simulink model "systema_script"  (R2019a)
settings: Solver=ode4  StartTime=0.0  StopTime=20  FixedStep=0.01  RelTol=1e-3  EnableMultiTasking=on
undefined symbols (not defined in the file or in its folder): dfod, DiscIntNeverNeededParam, f_enable, gain, i_enable, iokd, ioki, iokp, Kd, Kp, Lambda
libraries: simulink x9
settings Model: Creator=ece  LastModifiedBy=standard
settings DataIOCC: SaveFormat=Array  ReturnWorkspaceOutputs=off  SignalLoggingName=sigsOut
settings OptimizationCC: OptimizeBlockIOStorage=off  BufferReuse=off  GlobalBufferReuse=off  ExpressionFolding=off  ExpressionDepthLimit=2147483647  LocalBlockOutputs=off  InitFltsAndDblsToZero=on  LifeSpan=inf  OptimizeDataStoreBuffers=off  BusAssignmentInplaceUpdate=off
settings DebuggingCC: SaveWithParameterizedLinksMsg=none  UnderspecifiedInitializationDetection=Classic  MergeDetectMultiDrivingBlocksExec=none  SignalResolutionControl=TryResolveAllWithWarning  MultiTaskDSMMsg=warning  MultiTaskCondExecSysMsg=none  FcnCallInpInsideContextMsg=warning  StateNameClashWarn=warning  PregeneratedLibrarySubsystemCodeDiagnostic=none  SFUnexpectedBacktrackingDiag=warning  SFNoUnconditionalDefaultTransitionDiag=warning  SFExecutionAtInitializationDiag=none  ArithmeticOperatorsInVariantConditions=warning
settings HardwareCC: ProdBitPerPointer=32  ProdBitPerSizeT=32  ProdBitPerPtrDiffT=32  ProdLargestAtomicFloat=None  ProdIntDivRoundTo=Undefined  ProdEndianess=Unspecified  ProdWordSize=32  ProdHWDeviceType=32-bit Generic  TargetUnknown=on
settings ModelReferenceCC: PropagateSignalLabelsOutOfModel=off
settings SFSimCC: SimUseLocalCustomCode=off
settings RTWCC: RTWUseLocalCustomCode=off
settings CodeAppCC: StateflowObjectComments=on
settings GRTTargetCC: TargetFcnLib=ansi_tfl_tmw.mat  TargetLangStandard=C89/C90 (ANSI)  ModelReferenceCompliant=off  GeneratePreprocessorConditionals=Disable all  CombineOutputUpdateFcns=off  MatFileLogging=off  GRTInterface=on
settings ConfigComp: CovMetricSettings=dw  CovHtmlReporting=on  CovSaveCumulativeToWorkspaceVar=on  CovSaveSingleToWorkspaceVar=on  CovExternalEMLEnable=off

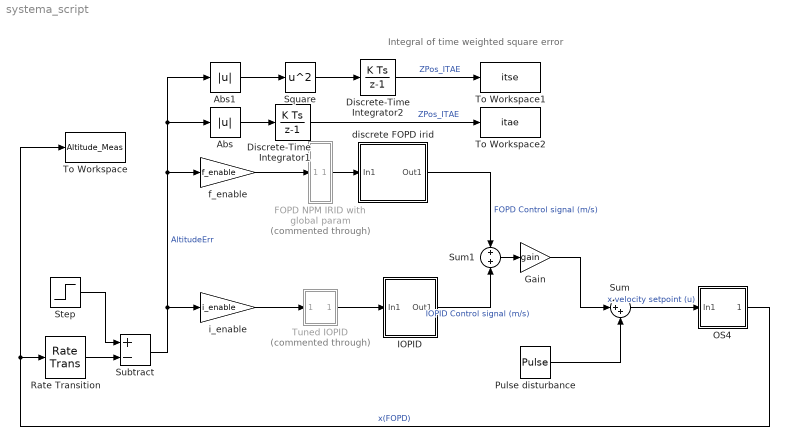
== system systema_script ==
  note: Integral of time weighted square error
  Abs : Abs
  Abs1 : Abs
  Discrete-Time Integrator1 : DiscreteIntegrator  SampleTime=-1  ICPrevOutput=DiscIntNeverNeededParam  ICPrevScaledInput=DiscIntNeverNeededParam
  Discrete-Time Integrator2 : DiscreteIntegrator  SampleTime=-1  ICPrevOutput=DiscIntNeverNeededParam  ICPrevScaledInput=DiscIntNeverNeededParam
  FOPD NPM IRID with global param : Subsystem  Commented=through
  Gain : Gain  Gain=gain
  IOPID : Subsystem
  OS4 : Subsystem
  Pulse disturbance : DiscretePulseGenerator  PulseType=Time based  Amplitude=0  Period=20  PhaseDelay=1
  Rate Transition : RateTransition  OutPortSampleTime=0.01
  Square : Math  Operator=square  SaturateOnIntegerOverflow=on
  Step : Step  Time=5  SampleTime=0.01
  Subtract : Sum  Inputs=+-
  Sum : Sum  Inputs=|++
  Sum1 : Sum  Inputs=+|+
  To Workspace : ToWorkspace  VariableName=Altitude_Meas  SaveFormat=Timeseries  SampleTime=-1
  To Workspace1 : ToWorkspace  VariableName=itse  SaveFormat=Timeseries  SampleTime=-1
  To Workspace2 : ToWorkspace  VariableName=itae  SaveFormat=Timeseries  SampleTime=-1
  Tuned IOPID : Subsystem  Commented=through
  discrete FOPD irid : Subsystem
  f_enable : Gain  Gain=f_enable
  i_enable : Gain  Gain=i_enable
  wires:
  IOPID/1(Out1) -> Sum1/2  "IOPID Control signal (m/s)"
  OS4/1(Out4) -> Rate Transition/1, To Workspace/1  "x(FOPD)"
  Step/1 -> Subtract/1
  discrete FOPD irid/1(Out1) -> Sum1/1  "FOPD Control signal (m/s)"
  Rate Transition/1 -> Subtract/2
  Pulse disturbance/1 -> Sum/2
  Sum/1 -> OS4/1(In1)  "x velocity setpoint (u)"
  Sum1/1 -> Gain/1
  f_enable/1 -> FOPD NPM IRID with global param/1(In1)
  i_enable/1 -> Tuned IOPID/1(In1)
  Gain/1 -> Sum/1
  Abs1/1 -> Square/1
  Subtract/1 -> i_enable/1, Abs/1, Abs1/1, f_enable/1  "AltitudeErr"
  Abs/1 -> Discrete-Time Integrator1/1
  Discrete-Time Integrator1/1 -> To Workspace2/1  "ZPos_ITAE"
  Square/1 -> Discrete-Time Integrator2/1
  Discrete-Time Integrator2/1 -> To Workspace1/1  "ZPos_ITAE"
  Tuned IOPID/1(Out1) -> IOPID/1(In1)
  FOPD NPM IRID with global param/1(Out1) -> discrete FOPD irid/1(In1)

== system systema_script/FOPD NPM IRID with global param ==
  note: FOPD controller
  In1 : Inport
  Discrete Transfer Fcn : DiscreteTransferFcn  Commented=through  Numerator=dfod.Num{1,1}  Denominator=dfod.Denominator{1,1}  SampleTime=0.01
  "Fractional operator " : Subsystem  Commented=through  mask{gam=Lambda, ww=[1e-3, 1e3], n=5, kF1=on, kF=Modified Oustaloup filter}
      mask prompts: gam "Derivative order gamma"; ww "Frequency range [wb,wh]"; n "Apprixmation order"; kF1 "Is a low-pass filter required?"; kF "Filter type"
      mask init:
      | wb=ww(1); wh=ww(2); 
      | if kF==1, G=ousta_fod(gam,n,wb,wh);
      | else, G=new_fod(gam,n,wb,wh); end
      | num=G.num{1}; den=G.den{1}; T=1/wh; str='Fractional\n';
      | if isnumeric(gam)
      | 	if gam>0, str=[str, 'Der  s^' num2str(gam) ];
      | 	else, str=[str, 'Int  s^{' num2str(gam) '}']; end
      | else, str=[str, 'Der  s^gam']; end
      | if kF1==1, G=G*tf(1,[T 1]); end
      mask TypeOptions kF: Oustaloup filter | Modified Oustaloup filter | Matsuda-Fujii filter
      mask Display: disp(str)
  Saturation : Saturate  UpperLimit=5  LowerLimit=-5
  Saturation1 : Saturate  UpperLimit=5  LowerLimit=-5
  Sum : Sum  Inputs=++|
  k_d : Gain  Gain=Kd
  k_p : Gain  Gain=Kp
  Out1 : Outport
  wires:
  In1/1 -> k_p/1  "P"
  Sum/1 -> Saturation1/1
  Saturation1/1 -> Out1/1
  k_d/1 -> "Fractional operator "/1(In1)  "DD_input"
  Discrete Transfer Fcn/1 -> Saturation/1  "DD_out"
  Saturation/1 -> Sum/2  "D"
  "Fractional operator "/1(Out1) -> Discrete Transfer Fcn/1
  k_p/1 -> Sum/1, k_d/1  "DD_input"

== system systema_script/IOPID ==
  In1 : Inport
  Discrete Derivative : simulink/Discrete/Discrete Derivative  gainval=1.0  ICPrevScaledInput=0.0  OutMin=[]  OutMax=[]  OutDataType=fixdt(1, 16)  OutScaling=2^-10  DoSatur=off
  Discrete-Time Integrator : DiscreteIntegrator  SampleTime=-1  ICPrevOutput=DiscIntNeverNeededParam  ICPrevScaledInput=DiscIntNeverNeededParam
  Gain : Gain  Gain=1.58
  Gain1 : Gain  Gain=0.182
  Gain2 : Gain  Gain=1.49
  Sum2 : Sum  Inputs=+++
  Out1 : Outport
  wires:
  In1/1 -> Gain/1, Gain2/1, Gain1/1
  Gain/1 -> Sum2/1
  Gain1/1 -> Discrete-Time Integrator/1
  Gain2/1 -> Discrete Derivative/1
  Sum2/1 -> Out1/1
  Discrete Derivative/1 -> Sum2/3
  Discrete-Time Integrator/1 -> Sum2/2

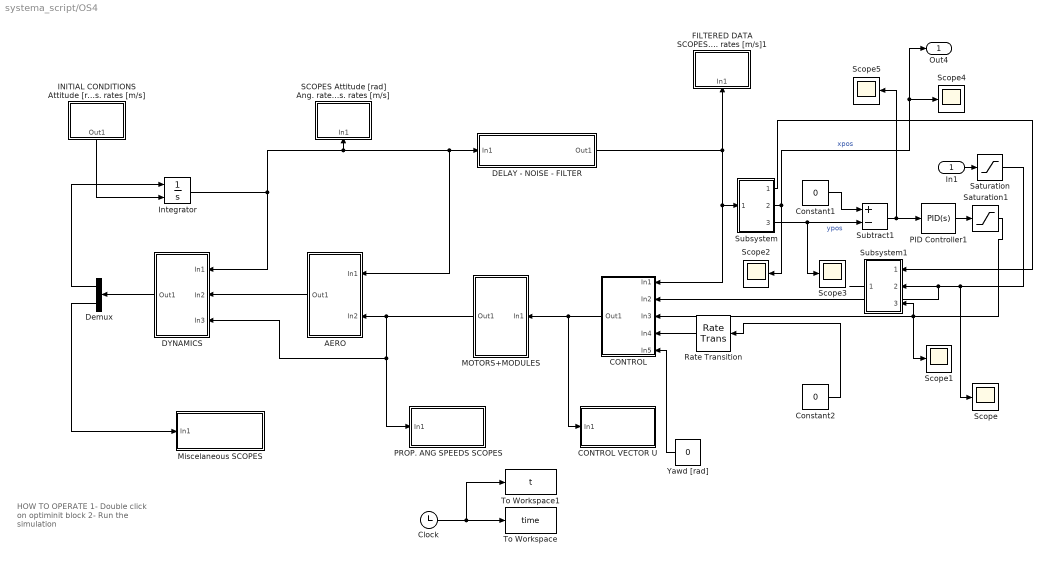
== system systema_script/OS4 ==
  note: HOW TO OPERATE
      | 1- Double click on optiminit block
      | 2- Run the simulation
  In1 : Inport
  AERO : Subsystem
  CONTROL : Subsystem
  CONTROL VECTOR U : Subsystem
  Clock : Clock
  Constant1 : Constant  Value=0
  Constant2 : Constant  Value=0
  DELAY - NOISE - FILTER : Subsystem
  DYNAMICS : Subsystem
  Demux : Demux  Outputs=2
  FILTERED DATA SCOPES Attitude [rad] Ang. rates [rad/sec] position [m] Pos. rates [m/s]1 : Subsystem
  "INITIAL CONDITIONS Attitude [rad] Ang. rates [rad/sec] position [m] Pos. rates [m/s] " : Subsystem
  Integrator : Integrator  InitialConditionSource=external
  MOTORS+MODULES : Subsystem
  Miscelaneous SCOPES : Subsystem
  PID Controller1 : simulink/Continuous/PID Controller  Controller=PID  Form=Parallel  TimeDomain=Continuous-time  SampleTime=-1  IntegratorMethod=Forward Euler  FilterMethod=Forward Euler  ControllerParametersSource=internal  P=1  I=0.2  D=0  UseFilter=on  N=100  TunerSelectOption=Transfer Function Based (PID Tuner App)  InitialConditionSource=internal  InitialConditionForIntegrator=0  InitialConditionForFilter=0  DifferentiatorICPrevScaledInput=0  ExternalReset=none  TrackingMode=off  Kt=1  LimitOutput=off  UpperSaturationLimit=inf  LowerSaturationLimit=-inf  LinearizeAsGain=off  AntiWindupMode=none  Kb=1  POutMin=[]  POutMax=[]  IOutMin=[]  IOutMax=[]  DOutMin=[]  DOutMax=[]  NOutMin=[]  NOutMax=[]  SumOutMin=[]  SumOutMax=[]  SaturationOutMin=[]  SaturationOutMax=[]  PParamMin=[]  PParamMax=[]  IParamMin=[]  IParamMax=[]  DParamMin=[]  DParamMax=[]  NParamMin=[]  NParamMax=[]  KbParamMin=[]  KbParamMax=[]  KtParamMin=[]  KtParamMax=[]  KbOutMin=[]  KbOutMax=[]  KtOutMin=[]  KtOutMax=[]  IntegratorOutMin=[]  IntegratorOutMax=[]  FilterOutMin=[]  FilterOutMax=[]  SumI1OutMin=[]  SumI1OutMax=[]  SumI2OutMin=[]  SumI2OutMax=[]  SumI3OutMin=[]  SumI3OutMax=[]  SumI4OutMin=[]  SumI4OutMax=[]  SumDOutMin=[]  SumDOutMax=[]  DifferentiatorOutMin=[]  DifferentiatorOutMax=[]  FilterDiffOutCoefMin=[]  FilterDiffOutCoefMax=[]  ReciprocalOutMin=[]  ReciprocalOutMax=[]  SumDenOutMin=[]  SumDenOutMax=[]  SumNumOutMin=[]  SumNumOutMax=[]  DivideOutMin=[]  DivideOutMax=[]  IntegratorContinuousStateAttributes=''  IntegratorStateMustResolveToSignalObject=off  IntegratorRTWStateStorageClass=Auto  FilterContinuousStateAttributes=''  FilterStateMustResolveToSignalObject=off  FilterRTWStateStorageClass=Auto  ParallelPVariant=InternalParameters  IdealPVariant=Disabled  IVariant=InternalParameters  DVariant=InternalParameters  IntegratorVariant=Continuous  SatVariant=Disabled  AWVariant=Passthrough  PCopyVariant=Disabled  TRVariant=Disabled  FdbkBlocksVariant=Forward  IdealPFdbkVariant=Disabled  SatFdbkVariant=Disabled  DerivativeFilterVariant=ContFilter  NVariant=InternalParameters  NCopyVariant=Disabled  FilterICVariant=InternalICsFilter  IntegratorICVariant=InternalICs  ExternalResetVariant=Disabled  TRSumVariant=Passthrough  SumFdbkVariant=Disabled  SumVariant=Sum_PID
  PROP. ANG SPEEDS SCOPES : Subsystem
  Rate Transition : RateTransition
  SCOPES Attitude [rad] Ang. rates [rad/sec] position [m] Pos. rates [m/s] : Subsystem
  Saturation : Saturate  UpperLimit=20  LowerLimit=-20
  Saturation1 : Saturate  UpperLimit=20  LowerLimit=-20
  Scope{,1..5} (6 alike) : Scope
  Subsystem : Subsystem
  Subsystem1 : Subsystem
  Subtract1 : Sum  Inputs=+-
  To Workspace : ToWorkspace  VariableName=time  SampleTime=-1
  To Workspace1 : ToWorkspace  VariableName=t  SampleTime=-1
  Yawd [rad] : Constant  Value=0
  Out4 : Outport
  wires:
  Demux/2 -> Miscelaneous SCOPES/1(In1)
  Integrator/1 -> SCOPES Attitude [rad] Ang. rates [rad/sec] position [m] Pos. rates [m/s]/1(In1), DELAY - NOISE - FILTER/1(In1), AERO/1(In1), DYNAMICS/1(In1)
  MOTORS+MODULES/1(Out1) -> AERO/2(In2), DYNAMICS/3(In3), PROP. ANG SPEEDS SCOPES/1(In1)
  Rate Transition/1 -> CONTROL/4(In4)
  CONTROL/1(Out1) -> MOTORS+MODULES/1(In1), CONTROL VECTOR U/1(In1)
  Yawd [rad]/1 -> CONTROL/5(In5)
  Constant2/1 -> Rate Transition/1
  Subsystem/2(Out3) -> Out4/1, Scope4/1, Scope2/1  "xpos"
  DELAY - NOISE - FILTER/1(Out1) -> FILTERED DATA SCOPES Attitude [rad] Ang. rates [rad/sec] position [m] Pos. rates [m/s]1/1(In1), CONTROL/1(In1), Subsystem/1(In1)
  Saturation1/1 -> CONTROL/3(In3), Subsystem1/3(In3), Scope1/1
  Saturation/1 -> Scope/1, Subsystem1/2(In2), CONTROL/2(In2)
  Subtract1/1 -> PID Controller1/1, Scope5/1
  Constant1/1 -> Subtract1/1
  Subsystem/1(Out2) -> Subsystem1/1(In1)
  PID Controller1/1 -> Saturation1/1
  Subsystem1/1(Out5) -> ?
  Subsystem/3(Out4) -> Subtract1/2, Scope3/1  "ypos"
  DYNAMICS/1(Out1) -> Demux/1
  In1/1 -> Saturation/1
  AERO/1(Out1) -> DYNAMICS/2(In2)
  "INITIAL CONDITIONS Attitude [rad] Ang. rates [rad/sec] position [m] Pos. rates [m/s] "/1(Out1) -> Integrator/2
  Clock/1 -> To Workspace/1, To Workspace1/1
  Demux/1 -> Integrator/1

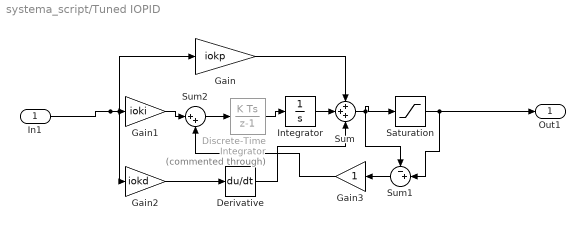
== system systema_script/Tuned IOPID ==
  In1 : Inport
  Derivative : Derivative
  Discrete-Time Integrator : DiscreteIntegrator  Commented=through  SampleTime=-1  ICPrevOutput=DiscIntNeverNeededParam  ICPrevScaledInput=DiscIntNeverNeededParam
  Gain : Gain  Gain=iokp
  Gain1 : Gain  Gain=ioki
  Gain2 : Gain  Gain=iokd
  Gain3 : Gain
  Integrator : Integrator
  Saturation : Saturate  UpperLimit=10  LowerLimit=-10
  Sum : Sum  Inputs=+++
  Sum1 : Sum  Inputs=-+|
  Sum2 : Sum  Inputs=|++
  Out1 : Outport
  wires:
  Sum/1 -> Saturation/1, Sum1/1
  Sum1/1 -> Gain3/1
  In1/1 -> Gain2/1, Gain/1, Gain1/1
  Sum2/1 -> Discrete-Time Integrator/1
  Derivative/1 -> Sum/3
  Gain/1 -> Sum/1
  Discrete-Time Integrator/1 -> Integrator/1
  Gain1/1 -> Sum2/1
  Gain3/1 -> Sum2/2
  Gain2/1 -> Derivative/1
  Saturation/1 -> Sum1/2, Out1/1
  Integrator/1 -> Sum/2

== system systema_script/discrete FOPD irid ==
  In1 : Inport
  Discrete Transfer Fcn : DiscreteTransferFcn  Numerator=[1,-3.83915008336134,5.68830152517571,-4.01123857485582,1.31417664909109,-0.152089532241851]  Denominator=[8.08505564819526e-05,-0.000204449367025327,0.000263365621479140,-0.000214834792194125,8.91860440440781e-05,-1.22283037538058e-05]
  Discrete-Time Integrator : DiscreteIntegrator  SampleTime=-1  ICPrevOutput=DiscIntNeverNeededParam  ICPrevScaledInput=DiscIntNeverNeededParam
  Gain : Gain  Gain=1.5489
  Gain1 : Gain  Gain=0.8829
  Sum : Sum  Inputs=|++
  Out1 : Outport
  wires:
  Sum/1 -> Out1/1  "vx set"
  In1/1 -> Gain/1  "x err"
  Gain/1 -> Gain1/1, Sum/1
  Gain1/1 -> Discrete Transfer Fcn/1
  Discrete Transfer Fcn/1 -> Discrete-Time Integrator/1
  Discrete-Time Integrator/1 -> Sum/2

== system systema_script/FOPD NPM IRID with global param/Fractional operator  ==
  In1 : Inport
  Transfer Fcn : TransferFcn  Numerator=num  Denominator=den
  Out1 : Outport
  wires:
  In1/1 -> Transfer Fcn/1
  Transfer Fcn/1 -> Out1/1

== system systema_script/OS4/AERO ==
  In1 : Inport
  In2 : Inport  Port=2
  AERO Attitude [rad] : MATLABFcn  MATLABFcn=aero  OutputDimensions=24
  Mux1 : Mux  Inputs=2
  Out1 : Outport
  wires:
  In1/1 -> Mux1/1
  In2/1 -> Mux1/2
  Mux1/1 -> AERO Attitude [rad]/1
  AERO Attitude [rad]/1 -> Out1/1

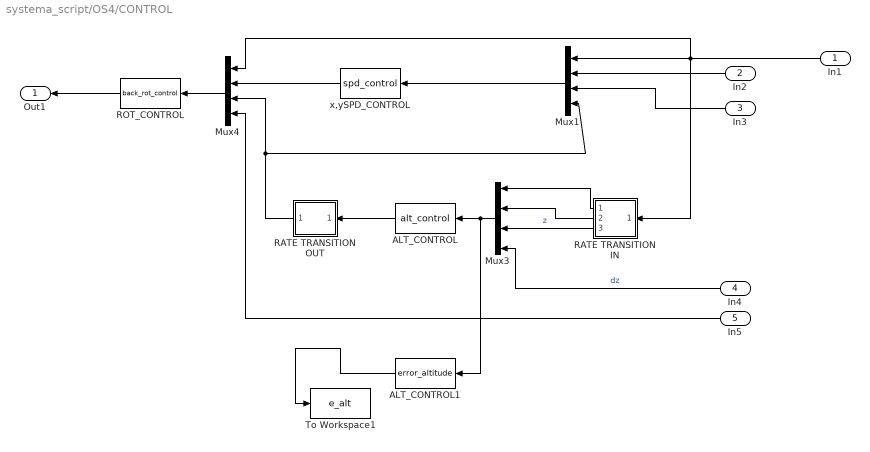
== system systema_script/OS4/CONTROL ==
  In1 : Inport
  In2 : Inport  Port=2
  In3 : Inport  Port=3
  In4 : Inport  Port=4
  In5 : Inport  Port=5
  ALT_CONTROL : MATLABFcn  MATLABFcn=alt_control  OutputDimensions=1  SampleTime=0.05
  ALT_CONTROL1 : MATLABFcn  MATLABFcn=error_altitude  OutputDimensions=1  SampleTime=0.05
  Mux1 : Mux
  Mux3 : Mux
  Mux4 : Mux
  RATE TRANSITION IN : Subsystem
  RATE TRANSITION OUT : Subsystem
  ROT_CONTROL : MATLABFcn  MATLABFcn=back_rot_control  OutputDimensions=6
  To Workspace1 : ToWorkspace  VariableName=e_alt  SampleTime=-1
  x,ySPD_CONTROL : MATLABFcn  MATLABFcn=spd_control  OutputDimensions=2
  Out1 : Outport
  wires:
  Mux1/1 -> x,ySPD_CONTROL/1
  ROT_CONTROL/1 -> Out1/1
  In1/1 -> Mux1/1, RATE TRANSITION IN/1(In1), Mux4/1
  In2/1 -> Mux1/2
  x,ySPD_CONTROL/1 -> Mux4/2
  Mux4/1 -> ROT_CONTROL/1
  ALT_CONTROL/1 -> RATE TRANSITION OUT/1(In1)
  In5/1 -> Mux4/4
  RATE TRANSITION OUT/1(Out1) -> Mux4/3, Mux1/4
  Mux3/1 -> ALT_CONTROL/1, ALT_CONTROL1/1
  RATE TRANSITION IN/1(Out1) -> Mux3/1
  RATE TRANSITION IN/2(Out2) -> Mux3/2
  RATE TRANSITION IN/3(Out3) -> Mux3/3  "z"
  In4/1 -> Mux3/4  "dz"
  In3/1 -> Mux1/3
  ALT_CONTROL1/1 -> To Workspace1/1

== system systema_script/OS4/CONTROL VECTOR U ==
  In1 : Inport
  Demux1 : Demux  Outputs=6
  U{1..4} (4 alike) : Scope
  e1 : Scope
  e2 : Scope
  wires:
  In1/1 -> Demux1/1
  Demux1/4 -> U4/1
  Demux1/3 -> U3/1
  Demux1/2 -> U2/1
  Demux1/1 -> U1/1
  Demux1/5 -> e1/1
  Demux1/6 -> e2/1

== system systema_script/OS4/DELAY - NOISE - FILTER ==
  In1 : Inport
  DELAYS : Subsystem
  LP FILTER : MATLABFcn  MATLABFcn=sam5_filter  OutputDimensions=12  OutputSignalType=real
  NOISY DATA SCOPES Attitude [rad] Ang. rates [rad/sec] position [m] Pos. rates [m/s]1 : Subsystem
  W. NORMAL NOISE1 : Subsystem
  Out1 : Outport
  wires:
  In1/1 -> DELAYS/1(In1)
  DELAYS/1(Out1) -> NOISY DATA SCOPES Attitude [rad] Ang. rates [rad/sec] position [m] Pos. rates [m/s]1/1(In1), LP FILTER/1
  LP FILTER/1 -> Out1/1

== system systema_script/OS4/DYNAMICS ==
  In1 : Inport
  In2 : Inport  Port=2
  In3 : Inport  Port=3
  DYNAMICS : MATLABFcn  MATLABFcn=dinamica  OutputDimensions=18
  Mux1 : Mux  Inputs=3
  Out1 : Outport
  wires:
  DYNAMICS/1 -> Out1/1
  Mux1/1 -> DYNAMICS/1
  In2/1 -> Mux1/2
  In1/1 -> Mux1/1
  In3/1 -> Mux1/3

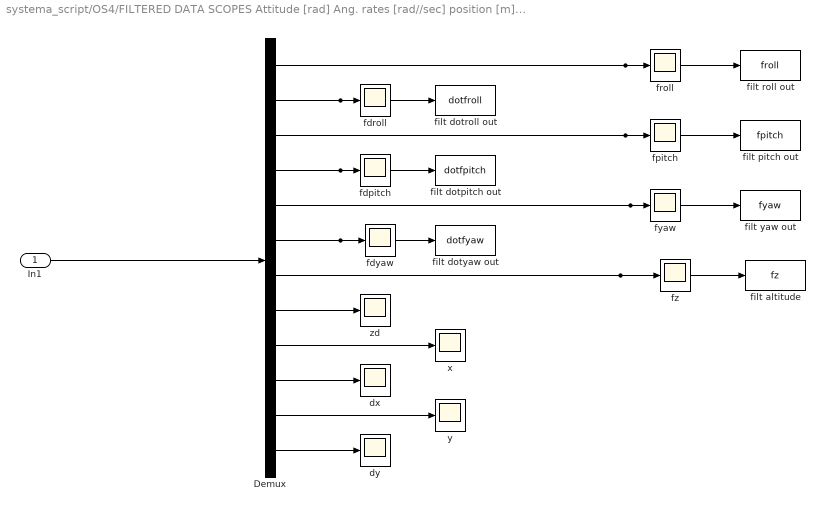
== system systema_script/OS4/FILTERED DATA SCOPES Attitude [rad] Ang. rates [rad//sec] position [m] Pos. rates [m//s]1 ==
  In1 : Inport
  Demux : Demux  Outputs=12
  dx : Scope
  dy : Scope
  fdpitch : Scope
  fdroll : Scope
  fdyaw : Scope
  filt altitude : ToWorkspace  VariableName=fz  SampleTime=-1
  filt dotpitch out : ToWorkspace  VariableName=dotfpitch  SampleTime=-1
  filt dotroll out : ToWorkspace  VariableName=dotfroll  SampleTime=-1
  filt dotyaw out : ToWorkspace  VariableName=dotfyaw  SampleTime=-1
  filt pitch out : ToWorkspace  VariableName=fpitch  SampleTime=-1
  filt roll out : ToWorkspace  VariableName=froll  SampleTime=-1
  filt yaw out : ToWorkspace  VariableName=fyaw  SampleTime=-1
  fpitch : Scope
  froll : Scope
  fyaw : Scope
  fz : Scope
  x : Scope
  y : Scope
  zd : Scope
  wires:
  Demux/1 -> filt roll out/1, froll/1
  Demux/4 -> fdpitch/1, filt dotpitch out/1
  Demux/8 -> zd/1
  Demux/7 -> filt altitude/1, fz/1
  Demux/6 -> fdyaw/1, filt dotyaw out/1
  Demux/2 -> fdroll/1, filt dotroll out/1
  Demux/5 -> filt yaw out/1, fyaw/1
  Demux/3 -> filt pitch out/1, fpitch/1
  In1/1 -> Demux/1
  Demux/9 -> x/1
  Demux/10 -> dx/1
  Demux/11 -> y/1
  Demux/12 -> dy/1

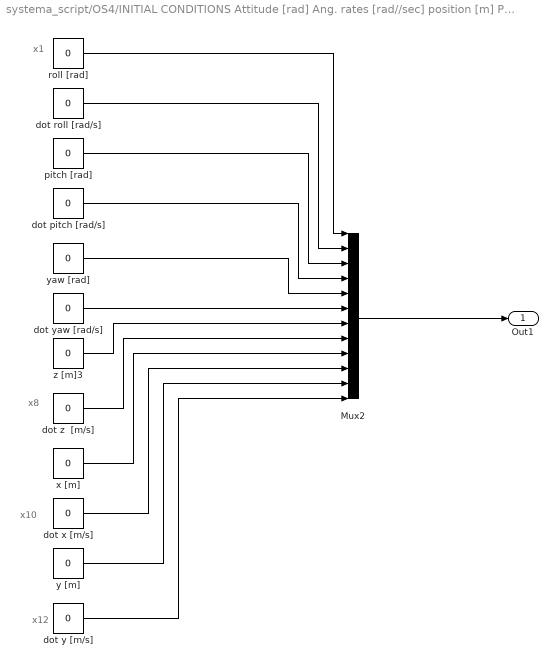
== system systema_script/OS4/INITIAL CONDITIONS Attitude [rad] Ang. rates [rad//sec] position [m] Pos. rates [m//s]  ==
  note: x1
  note: x12
  note: x10
  note: x8
  Mux2 : Mux  Inputs=12
  dot pitch [rad/s] : Constant  Value=0
  dot roll [rad/s] : Constant  Value=0
  dot x [m/s] : Constant  Value=0
  dot y [m/s] : Constant  Value=0
  dot yaw [rad/s] : Constant  Value=0
  dot z  [m/s] : Constant  Value=0
  pitch [rad] : Constant  Value=0
  roll [rad] : Constant  Value=0
  x [m] : Constant  Value=0
  y [m] : Constant  Value=0
  yaw [rad] : Constant  Value=0
  z [m]3 : Constant  Value=0
  Out1 : Outport
  wires:
  roll [rad]/1 -> Mux2/1
  dot roll [rad/s]/1 -> Mux2/2
  pitch [rad]/1 -> Mux2/3
  dot pitch [rad/s]/1 -> Mux2/4
  dot yaw [rad/s]/1 -> Mux2/6
  z [m]3/1 -> Mux2/7
  dot z  [m/s]/1 -> Mux2/8
  yaw [rad]/1 -> Mux2/5
  Mux2/1 -> Out1/1
  x [m]/1 -> Mux2/9
  dot x [m/s]/1 -> Mux2/10
  y [m]/1 -> Mux2/11
  dot y [m/s]/1 -> Mux2/12

== system systema_script/OS4/MOTORS+MODULES ==
  In1 : Inport
  Bin2Om : MATLABFcn  MATLABFcn=bin2Om  OutputDimensions=4  OutputSignalType=real
  MOTOR DYNAMICS : Subsystem
  Saturation : Saturate  UpperLimit=125  LowerLimit=10
  U2bin : MATLABFcn  MATLABFcn=U2bin  OutputDimensions=4  OutputSignalType=real
  Out1 : Outport
  wires:
  Bin2Om/1 -> Out1/1
  MOTOR DYNAMICS/1(Out1) -> Bin2Om/1
  U2bin/1 -> Saturation/1
  In1/1 -> U2bin/1
  Saturation/1 -> MOTOR DYNAMICS/1(In1)

== system systema_script/OS4/Miscelaneous SCOPES ==
  In1 : Inport  PortDimensions=6
  Demux : Demux  Outputs=6
  raa : Scope
  rgb : Scope
  rgp : Scope
  rhf : Scope
  rrm : Scope
  rrm1 : Scope
  wires:
  In1/1 -> Demux/1
  Demux/5 -> rrm/1
  Demux/4 -> rhf/1
  Demux/3 -> raa/1
  Demux/2 -> rgp/1
  Demux/1 -> rgb/1
  Demux/6 -> rrm1/1

== system systema_script/OS4/PROP. ANG SPEEDS SCOPES ==
  In1 : Inport
  Demux1 : Demux
  omega{1..4} (4 alike) : Scope
  wires:
  Demux1/1 -> omega1/1
  Demux1/2 -> omega2/1
  Demux1/3 -> omega3/1
  Demux1/4 -> omega4/1
  In1/1 -> Demux1/1

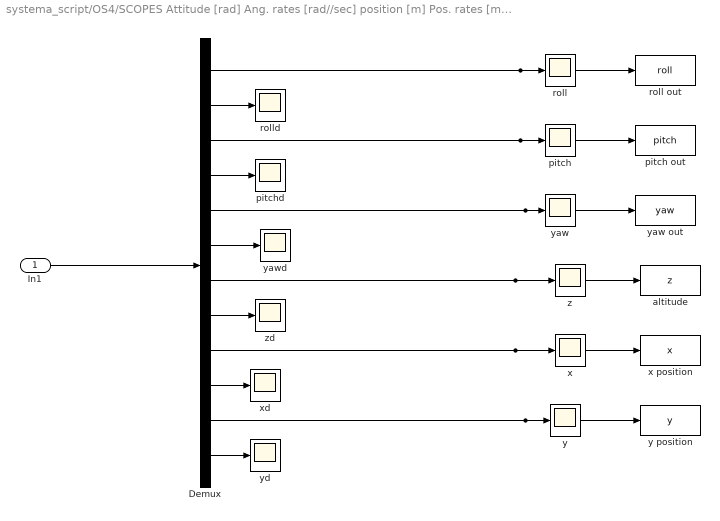
== system systema_script/OS4/SCOPES Attitude [rad] Ang. rates [rad//sec] position [m] Pos. rates [m//s] ==
  In1 : Inport
  Demux : Demux  Outputs=12
  altitude : ToWorkspace  VariableName=z  SampleTime=-1
  pitch : Scope
  pitch out : ToWorkspace  VariableName=pitch  SampleTime=-1
  pitchd : Scope
  roll : Scope
  roll out : ToWorkspace  VariableName=roll  SampleTime=-1
  rolld : Scope
  x : Scope
  x position : ToWorkspace  VariableName=x  SampleTime=-1
  xd : Scope
  y : Scope
  y position : ToWorkspace  VariableName=y  SampleTime=-1
  yaw : Scope
  yaw out : ToWorkspace  VariableName=yaw  SampleTime=-1
  yawd : Scope
  yd : Scope
  z : Scope
  zd : Scope
  wires:
  In1/1 -> Demux/1
  Demux/3 -> pitch/1, pitch out/1
  Demux/5 -> yaw/1, yaw out/1
  Demux/2 -> rolld/1
  Demux/6 -> yawd/1
  Demux/7 -> z/1, altitude/1
  Demux/8 -> zd/1
  Demux/9 -> x/1, x position/1
  Demux/11 -> y/1, y position/1
  Demux/12 -> yd/1
  Demux/10 -> xd/1
  Demux/4 -> pitchd/1
  Demux/1 -> roll/1, roll out/1

== system systema_script/OS4/Subsystem ==
  In1 : Inport
  Demux1 : Demux  Outputs=12
  Double click on this for demo.5 : Subsystem
      settings: OpenFcn=optsiminit
      mask Display: disp('optsiminit')
  Mux1 : Mux  Inputs=10
  Out2 : Outport
  Out3 : Outport  Port=2
  Out4 : Outport  Port=3
  wires:
  Demux1/1 -> Mux1/1
  Demux1/2 -> Mux1/2
  Demux1/3 -> Mux1/3
  Demux1/4 -> Mux1/4
  Demux1/5 -> Mux1/5
  Demux1/6 -> Mux1/6
  Demux1/7 -> Mux1/7
  Demux1/8 -> Mux1/8
  Demux1/10 -> Mux1/9
  Demux1/12 -> Mux1/10
  Mux1/1 -> Out2/1
  Demux1/9 -> Out3/1
  Demux1/11 -> Out4/1
  In1/1 -> Demux1/1

== system systema_script/OS4/Subsystem1 ==
  In1 : Inport
  In2 : Inport  Port=2
  In3 : Inport  Port=3
  Demux1 : Demux  Outputs=10
  Mux1 : Mux  Inputs=12
  Out5 : Outport
  wires:
  In1/1 -> Demux1/1
  Demux1/1 -> Mux1/1
  Demux1/2 -> Mux1/2
  Demux1/3 -> Mux1/3
  Demux1/4 -> Mux1/4
  Demux1/5 -> Mux1/5
  Demux1/6 -> Mux1/6
  Demux1/7 -> Mux1/7
  Demux1/8 -> Mux1/8
  Demux1/10 -> Mux1/12
  Demux1/9 -> Mux1/10
  In2/1 -> Mux1/9
  In3/1 -> Mux1/11
  Mux1/1 -> Out5/1

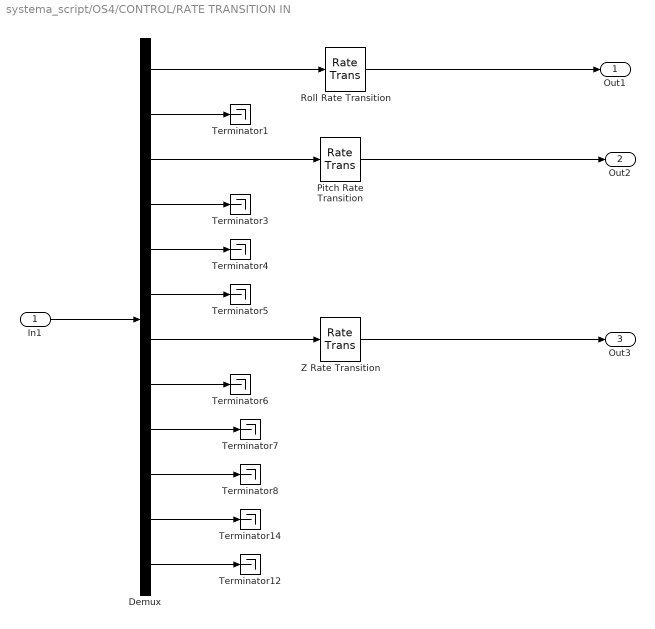
== system systema_script/OS4/CONTROL/RATE TRANSITION IN ==
  In1 : Inport
  Demux : Demux  Outputs=12
  Pitch Rate Transition : RateTransition  Deterministic=off  OutPortSampleTime=50E-3
  Roll Rate Transition : RateTransition  Deterministic=off  OutPortSampleTime=50E-3
  Terminator{1,3..8,12,14} (9 alike) : Terminator
  Z Rate Transition : RateTransition  Deterministic=off  OutPortSampleTime=50E-3
  Out1 : Outport
  Out2 : Outport  Port=2
  Out3 : Outport  Port=3
  wires:
  Demux/7 -> Z Rate Transition/1
  In1/1 -> Demux/1
  Demux/1 -> Roll Rate Transition/1
  Demux/2 -> Terminator1/1
  Demux/3 -> Pitch Rate Transition/1
  Demux/4 -> Terminator3/1
  Demux/5 -> Terminator4/1
  Demux/6 -> Terminator5/1
  Demux/9 -> Terminator7/1
  Demux/10 -> Terminator8/1
  Demux/11 -> Terminator14/1
  Demux/12 -> Terminator12/1
  Demux/8 -> Terminator6/1
  Roll Rate Transition/1 -> Out1/1
  Pitch Rate Transition/1 -> Out2/1
  Z Rate Transition/1 -> Out3/1

== system systema_script/OS4/CONTROL/RATE TRANSITION OUT ==
  In1 : Inport
  Rate Transition1 : RateTransition  Deterministic=off
  Out1 : Outport
  wires:
  In1/1 -> Rate Transition1/1
  Rate Transition1/1 -> Out1/1

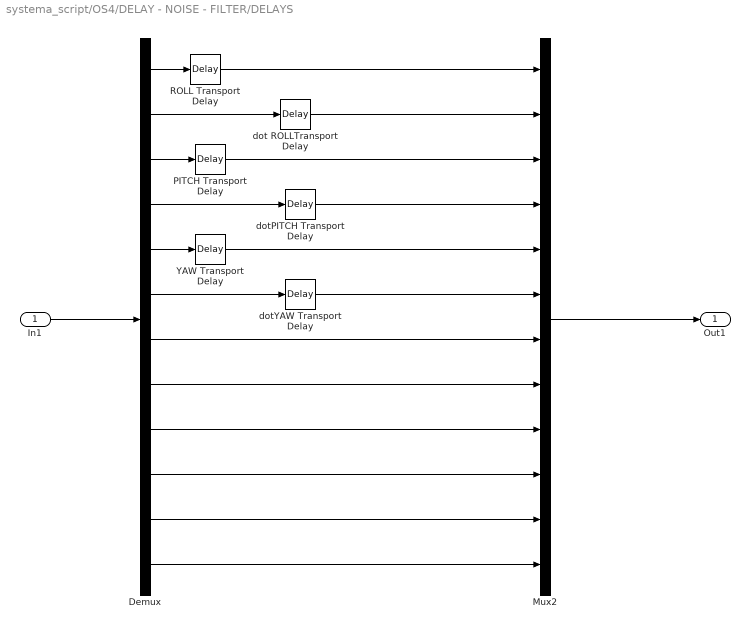
== system systema_script/OS4/DELAY - NOISE - FILTER/DELAYS ==
  In1 : Inport
  Demux : Demux  Outputs=12
  Mux2 : Mux  Inputs=12
  PITCH Transport Delay : TransportDelay  DelayTime=8E-3
  ROLL Transport Delay : TransportDelay  DelayTime=8E-3
  YAW Transport Delay : TransportDelay  DelayTime=8E-3
  dot ROLLTransport Delay : TransportDelay  DelayTime=4.5E-3
  dotPITCH Transport Delay : TransportDelay  DelayTime=4.5E-3
  dotYAW Transport Delay : TransportDelay  DelayTime=4.5E-3
  Out1 : Outport
  wires:
  dot ROLLTransport Delay/1 -> Mux2/2
  Demux/12 -> Mux2/12
  Demux/11 -> Mux2/11
  Demux/10 -> Mux2/10
  Demux/9 -> Mux2/9
  Demux/8 -> Mux2/8
  Demux/7 -> Mux2/7
  dotYAW Transport Delay/1 -> Mux2/6
  Demux/6 -> dotYAW Transport Delay/1
  YAW Transport Delay/1 -> Mux2/5
  Demux/5 -> YAW Transport Delay/1
  dotPITCH Transport Delay/1 -> Mux2/4
  Demux/4 -> dotPITCH Transport Delay/1
  PITCH Transport Delay/1 -> Mux2/3
  Demux/3 -> PITCH Transport Delay/1
  Demux/2 -> dot ROLLTransport Delay/1
  ROLL Transport Delay/1 -> Mux2/1
  Demux/1 -> ROLL Transport Delay/1
  In1/1 -> Demux/1
  Mux2/1 -> Out1/1

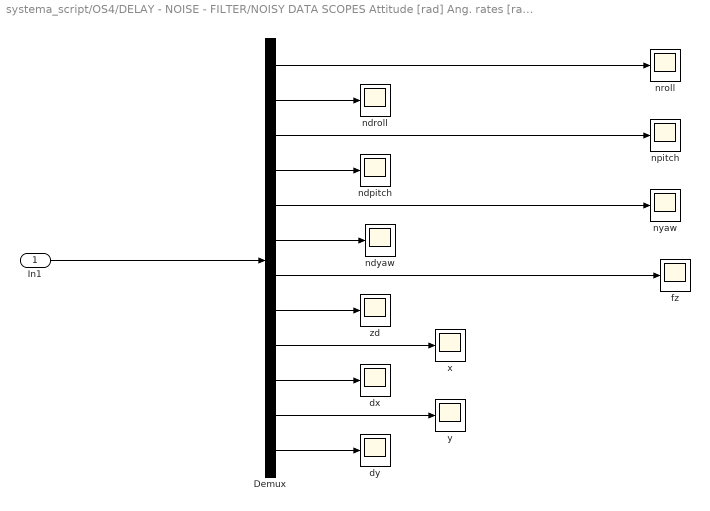
== system systema_script/OS4/DELAY - NOISE - FILTER/NOISY DATA SCOPES Attitude [rad] Ang. rates [rad//sec] position [m] Pos. rates [m//s]1 ==
  In1 : Inport
  Demux : Demux  Outputs=12
  dx : Scope
  dy : Scope
  fz : Scope
  ndpitch : Scope
  ndroll : Scope
  ndyaw : Scope
  npitch : Scope
  nroll : Scope
  nyaw : Scope
  x : Scope
  y : Scope
  zd : Scope
  wires:
  Demux/1 -> nroll/1
  Demux/4 -> ndpitch/1
  Demux/8 -> zd/1
  Demux/7 -> fz/1
  Demux/6 -> ndyaw/1
  Demux/2 -> ndroll/1
  Demux/5 -> nyaw/1
  Demux/3 -> npitch/1
  In1/1 -> Demux/1
  Demux/9 -> x/1
  Demux/10 -> dx/1
  Demux/11 -> y/1
  Demux/12 -> dy/1

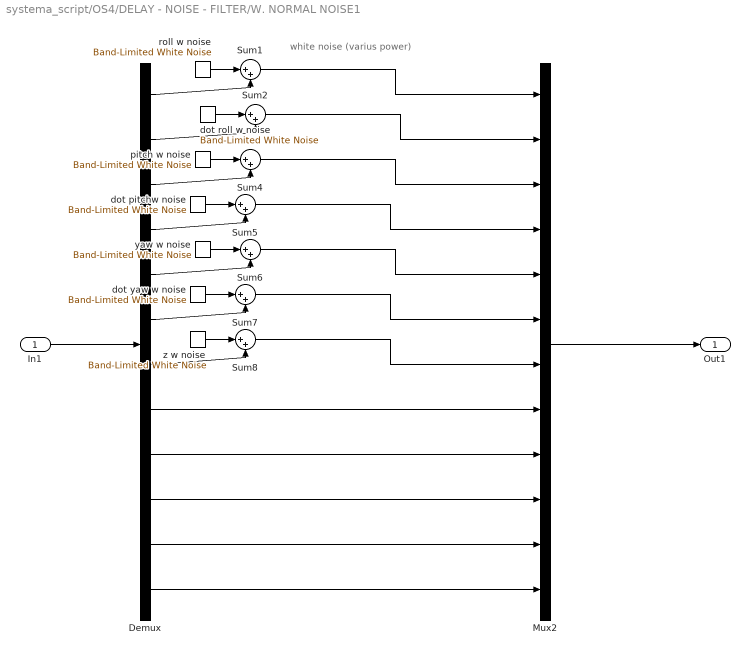
== system systema_script/OS4/DELAY - NOISE - FILTER/W. NORMAL NOISE1 ==
  note: white noise (varius power)
  In1 : Inport
  Demux : Demux  Outputs=12
  Mux2 : Mux  Inputs=12
  Sum{1..2,4..8} (7 alike) : Sum  Inputs=|++  SaturateOnIntegerOverflow=on
  dot pitchw noise : simulink/Sources/Band-Limited White Noise  Cov=[0.0001]  Ts=0.01  seed=[23341]
  dot roll w noise : simulink/Sources/Band-Limited White Noise  Cov=[0.0001]  Ts=0.01  seed=[23341]
  dot yaw w noise : simulink/Sources/Band-Limited White Noise  Cov=[0.0001]  Ts=0.01  seed=[23341]
  pitch w noise : simulink/Sources/Band-Limited White Noise  Cov=[0.00001]  Ts=0.01  seed=[23341]
  roll w noise : simulink/Sources/Band-Limited White Noise  Cov=[0.00001]  Ts=0.01  seed=[24431]
  yaw w noise : simulink/Sources/Band-Limited White Noise  Cov=[0.00001]  Ts=0.01  seed=[23341]
  z w noise : simulink/Sources/Band-Limited White Noise  Cov=[0.00001]  Ts=0.01  seed=[23341]
  Out1 : Outport
  wires:
  Demux/8 -> Mux2/8
  Demux/12 -> Mux2/12
  Demux/11 -> Mux2/11
  Demux/10 -> Mux2/10
  Demux/9 -> Mux2/9
  Sum8/1 -> Mux2/7
  z w noise/1 -> Sum8/1
  Demux/7 -> Sum8/2
  Sum7/1 -> Mux2/6
  dot yaw w noise/1 -> Sum7/1
  Demux/6 -> Sum7/2
  Sum6/1 -> Mux2/5
  yaw w noise/1 -> Sum6/1
  Demux/5 -> Sum6/2
  Sum5/1 -> Mux2/4
  dot pitchw noise/1 -> Sum5/1
  Demux/4 -> Sum5/2
  Sum4/1 -> Mux2/3
  pitch w noise/1 -> Sum4/1
  Demux/3 -> Sum4/2
  Sum2/1 -> Mux2/2
  dot roll w noise/1 -> Sum2/1
  Demux/2 -> Sum2/2
  Sum1/1 -> Mux2/1
  roll w noise/1 -> Sum1/1
  Mux2/1 -> Out1/1
  In1/1 -> Demux/1
  Demux/1 -> Sum1/2

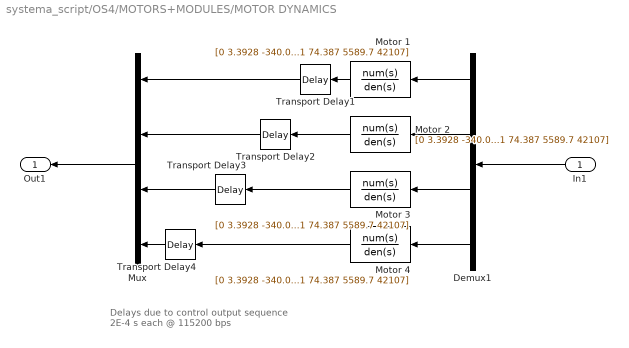
== system systema_script/OS4/MOTORS+MODULES/MOTOR DYNAMICS ==
  note: Delays due to control output sequence
      | 2E-4 s each @ 115200 bps
  In1 : Inport
  Demux1 : Demux
  Motor {1..4} (4 alike) : TransferFcn  Numerator=[0 3.3928 -340.09 39451]  Denominator=[1 74.387 5589.7 42107]
  Mux : Mux
  Transport Delay1 : TransportDelay  DelayTime=2E-4
  Transport Delay2 : TransportDelay  DelayTime=4E-4
  Transport Delay3 : TransportDelay  DelayTime=6E-4
  Transport Delay4 : TransportDelay  DelayTime=8E-4
  Out1 : Outport
  wires:
  In1/1 -> Demux1/1
  Demux1/1 -> Motor 1/1
  Demux1/2 -> Motor 2/1
  Demux1/3 -> Motor 3/1
  Demux1/4 -> Motor 4/1
  Motor 1/1 -> Transport Delay1/1
  Motor 2/1 -> Transport Delay2/1
  Motor 3/1 -> Transport Delay3/1
  Motor 4/1 -> Transport Delay4/1
  Mux/1 -> Out1/1
  Transport Delay2/1 -> Mux/2
  Transport Delay3/1 -> Mux/3
  Transport Delay4/1 -> Mux/4
  Transport Delay1/1 -> Mux/1

== system systema_script/OS4/Subsystem/Double click on this for demo.5 ==
